simulink model "testmodel"  (R2013a)
settings: Solver=ode45  StartTime=0.0  StopTime=25000  MaxStep=1  RelTol=1e-3
settings Model: Creator=johanneskazantzidis  LastModifiedBy=johanneskazantzidis
settings DebuggingCC: SolverPrmCheckMsg=none

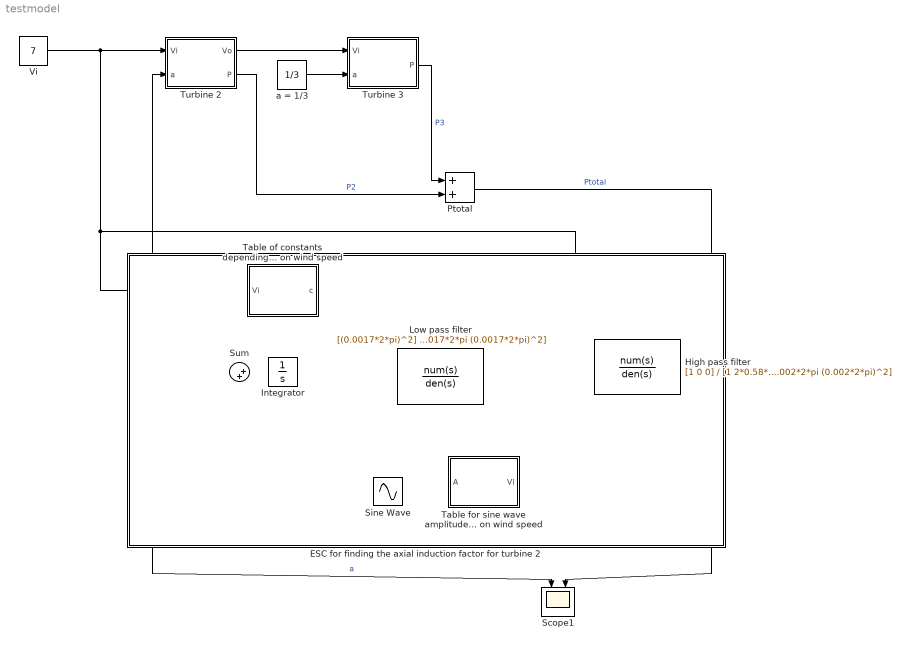
== system testmodel ==
  " " : Product
  "  " : Product
  "   " : Product
  "    " : Abs
  ESC for finding the axial induction factor for turbine 2 : Subsystem
  High pass filter : TransferFcn  Numerator=[1 0 0]  Denominator=[1 2*0.58*0.002*2*pi (0.002*2*pi)^2]
  Integrator : Integrator
  Low pass filter : TransferFcn  Numerator=[(0.0017*2*pi)^2]  Denominator=[1 2*0.6*0.0017*2*pi (0.0017*2*pi)^2]
  Ptotal : Sum
  Scope1 : Scope  NumInputPorts=2
      settings: ShowLegends=on  TimeRange=40000  YMin=0~2e+06  YMax=0.45~2.3e+06  MaxDataPoints=200000
  Sine Wave : Sin  SampleTime=0
  Sum : Sum  Inputs=|++
  Table for sine wave amplitudes depending on wind speed : MATLAB Function  TreatAsAtomicUnit=on
  Table of constants depending on wind speed : MATLAB Function  TreatAsAtomicUnit=on
  Turbine 2 : MATLAB Function  TreatAsAtomicUnit=on
  Turbine 3 : MATLAB Function  TreatAsAtomicUnit=on
  Vi : Constant  Value=7
  a = 1/3 : Constant  Value=1/3
  wires:
  Integrator/1 -> Sum/1
  "  "/1 -> Integrator/1
  Vi/1 -> Table of constants depending on wind speed/1(Vi), Table for sine wave amplitudes depending on wind speed/1(Vi), Turbine 2/1(Vi)
  High pass filter/1 -> " "/1
  "    "/1 -> Turbine 2/2(a), Scope1/1  "a"
  Turbine 2/2(P) -> Ptotal/2  "P2"
  Turbine 3/1(P) -> Ptotal/1  "P3"
  Turbine 2/1(Vo) -> Turbine 3/1(Vi)
  Ptotal/1 -> High pass filter/1, Scope1/2  "Ptotal"
  a = 1/3/1 -> Turbine 3/2(a)
  Low pass filter/1 -> "  "/2
  " "/1 -> Low pass filter/1
  Table for sine wave amplitudes depending on wind speed/1(A) -> "   "/2
  Sine Wave/1 -> "   "/1
  Table of constants depending on wind speed/1(c) -> "  "/1
  "   "/1 -> Sum/2, " "/2
  Sum/1 -> "    "/1

== system testmodel/ESC for finding the axial induction factor for turbine 2 ==

== matlab function testmodel/Turbine 2 ==
  data: Vo output; Vi input; P output; a input
function [ Vo, P] = turbineOut( Vi, a )
%UNTITLED2 Summary of this function goes here
%   Detailed explanation goes here
%% Check feasability
CI = 3.5; % Cut-in speed
CO = 26; % Cut-out speed

if Vi < CI
    Vo = 0;
    P = 0;
    return
elseif  Vi > CO
    Vo = 0;
    P = 0;
    return
else
    %% Declarations
    R = 75; % Blade radius m
    rho = 1.225; % Air density kg/m³
    Prated = 6e6; % Generation capability MW
    d = 500; % Distance in m between this turbine and the next. d is both the
    % (yu-yd) and (xu-xd) which is the distance between upstream and
    % downstream turbines (used for the gamma OF overlap factor
    
    
    %% Calculate power- and wind output
    Pwind = (1/2)*rho*pi*R.^2*Vi.^3;
    Cp = 4*a.*(1-a).^2;
    P = Pwind*Cp;
    P = min(P, Prated);
    
    
    Dc = 0.075; % Wake-decay constant. Determined empirically;
    gammaOF = (2*R+d*Dc)/R; % Overlap factor   2R+Dcd
    Ct = 4*a.*(1-a); % Turbine's thrust coefficient
    dV = Vi*(1-sqrt(1-Ct))*((2*R)/(2*R+2*Dc*d)).^2*gammaOF; % Velocity deficit
    
    Vo = max(Vi-dV, 0);
end

== matlab function testmodel/Turbine 3 ==
  data: Vi input; P output; a input
function P  = turbineOut( Vi, a )
%UNTITLED2 Summary of this function goes here
%   Detailed explanation goes here
%% Check feasability
CI = 3.5; % Cut-in speed
CO = 26; % Cut-out speed

if Vi < CI
    Vo = 0;
    P = 0;
    return
elseif  Vi > CO
    Vo = 0;
    P = 0;
    return
else
    %% Declarations
    R = 75; % Blade radius m
    rho = 1.225; % Air density kg/m³
    Prated = 6e6; % Generation capability MW
    d = 500; % Distance in m between this turbine and the next. d is both the
    % (yu-yd) and (xu-xd) which is the distance between upstream and
    % downstream turbines (used for the gamma OF overlap factor
    
    
    %% Calculate power
    % Note that wind output is irrelevant since this is the last turbine.
    Pwind = (1/2)*rho*pi*R.^2*Vi.^3;
    Cp = 4*a.*(1-a).^2;
    P = Pwind*Cp; 
    P = min(P, Prated);
    
    Dc = 0.075; % Wake-decay constant. Determined empirically;
    gammaOF = (2*R+d*Dc)/R; % Overlap factor   2R+Dcd
    Ct = 4*a.*(1-a); % Turbine's thrust coefficient
    dV = Vi*(1-sqrt(1-Ct))*((2*R)/(2*R+2*Dc*d)).^2*gammaOF; % Velocity deficit
    
    Vo = max(Vi-dV, 0);
end

== matlab function testmodel/Table for sine wave amplitudes depending on wind speed ==
  data: A output; Vi input
function A = Amplitude( Vi )
%UNTITLED2 Summary of this function goes here
%   Detailed explanation goes here
if Vi<=6.5
    A = 2e-3;
elseif Vi>6.5 && Vi<=7.5
A = 0.7e-3;
elseif Vi>12.5
    A = 4.5e-3;
elseif Vi>11.5 && Vi<=12.5
    A = 4e-3;
elseif Vi>10.5 && Vi<=11.5
    A = 7e-3;
elseif Vi>8.5 && Vi<=10.5
    A = 5e-3;
else
    A = 6e-3;
end
end

% function A = Amplitude( Vi )
% %UNTITLED2 Summary of this function goes here
% %   Detailed explanation goes here
% if Vi<=7.5
%     %A = 1.3e-3;
%     A = 0.7e-3;
% elseif Vi>12.5
%     A = 4.5e-3;
% elseif Vi>11.5 && Vi<=12.5
%     A = 4e-3;
% elseif Vi>10.5 && Vi<=11.5
%     A = 7e-3;
% elseif Vi>8.5 && Vi<=10.5
%     A = 5e-3;
% else
%     A = 6e-3;
% end
% end

== matlab function testmodel/Table of constants depending on wind speed ==
  data: c output; Vi input
function c   = delta( Vi )
%UNTITLED2 Summary of this function goes here
%   Detailed explanation goes here
if Vi<=6.5
    c = 8e-5;
elseif Vi>6.5 && Vi<7.5
    c = 8e-5;
elseif Vi>=12.5
    c = 3e-7;
elseif Vi>=10.5 && Vi<12.5
    c = 1e-7;
else
    c = 8e-6;
end
end

% function c   = delta( Vi )
% %UNTITLED2 Summary of this function goes here
% %   Detailed explanation goes here
% if Vi<=7.5
%     %c = 4e-5;
%     c = 8e-5;
% elseif Vi>=12.5
%     c = 3e-7;
% elseif Vi>=10.5 && Vi<12.5
%     c = 1e-7;
% else
%     c = 8e-6;
% end
% end
